simulink model "Solar_model2_AKhmad_Sameh"  (R2024b)
settings: Solver=FixedStepAuto  StartTime=0.0  StopTime=35000  FixedStep=1  RelTol=1e-3
settings Model: Creator=AKhmad  LastModifiedBy=AKhmad
settings OptimizationCC: ReuseModelBlockBuffer=off
settings RTWCC: GPUComputeCapability=3.5

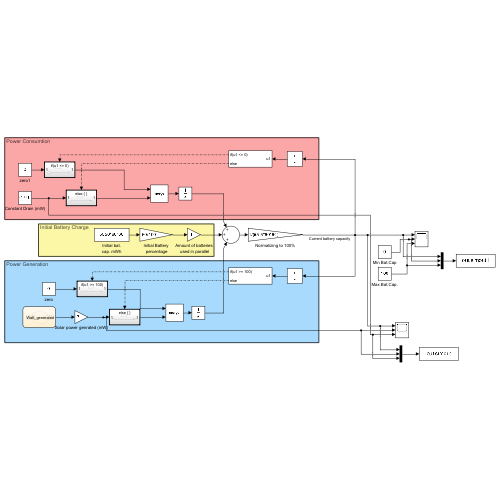
[thumbnail: Simulink's stored preview of the top-level diagram]
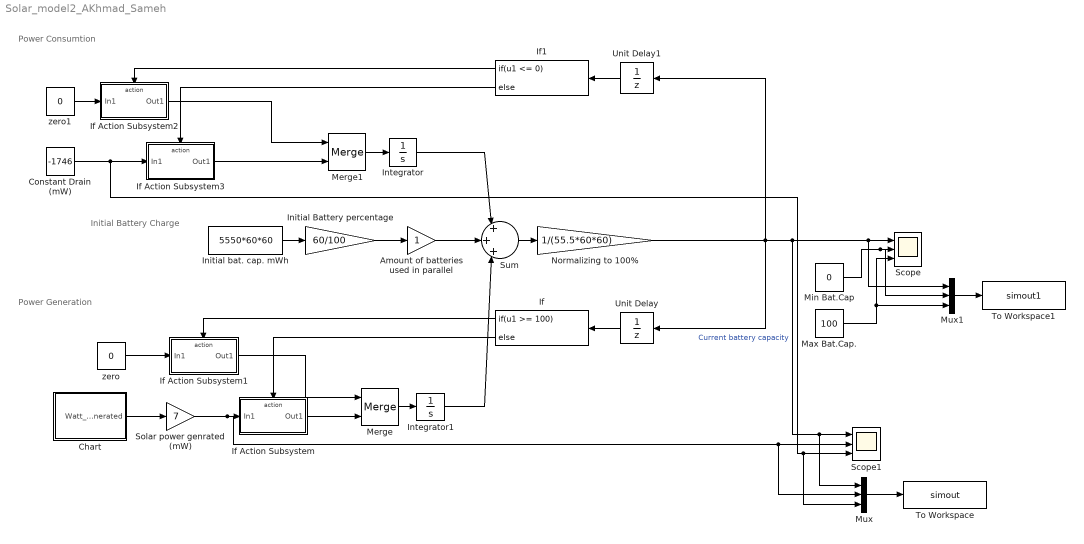
== system Solar_model2_AKhmad_Sameh ==
  note: Initial Battery Charge
  note: Power Generation
  note: Power Consumtion
  Amount of batteries used in parallel : Gain
  Chart : Stateflow chart  TreatAsAtomicUnit=on
  Constant Drain (mW) : Constant  Value=-1746
  If : If  IfExpression=u1 >= 100
  If Action Subsystem : Subsystem  TreatAsAtomicUnit=on
  If Action Subsystem1 : Subsystem  TreatAsAtomicUnit=on
  If Action Subsystem2 : Subsystem  TreatAsAtomicUnit=on
  If Action Subsystem3 : Subsystem  TreatAsAtomicUnit=on
  If1 : If  IfExpression=u1 <= 0
  Initial Battery percentage : Gain  Gain=60/100
  Initial bat. cap. mWh : Constant  Value=5550*60*60
  Integrator : Integrator
  Integrator1 : Integrator
  Max Bat.Cap. : Constant  Value=100
  Merge : Merge
  Merge1 : Merge
  Min Bat.Cap : Constant  Value=0
  Mux : Mux  Inputs=3
  Mux1 : Mux  Inputs=3
  Normalizing to 100% : Gain  Gain=1/(55.5*60*60)
  Scope : Scope  NumInputPorts=3
  Scope1 : Scope  NumInputPorts=3
  Solar power genrated (mW) : Gain  Gain=7
  Sum : Sum  Inputs=|+|+|+|  OutMin=0  OutMax=1
  To Workspace : ToWorkspace  VariableName=simout  SaveFormat=Timeseries  SampleTime=-1
  To Workspace1 : ToWorkspace  VariableName=simout1  SaveFormat=Timeseries  SampleTime=-1
  Unit Delay : UnitDelay  InitialCondition=100  SampleTime=-1  HasFrameUpgradeWarning=on
  Unit Delay1 : UnitDelay  InitialCondition=50  SampleTime=-1  HasFrameUpgradeWarning=on
  zero : Constant  Value=0
  zero1 : Constant  Value=0
  wires:
  Constant Drain (mW)/1 -> Mux/3, Scope1/3, If Action Subsystem3/1(In1)
  Integrator/1 -> Sum/1
  Chart/1(Watt_generated) -> Solar power genrated (mW)/1
  Sum/1 -> Normalizing to 100%/1
  Min Bat.Cap/1 -> Mux1/2, Scope/2
  Max Bat.Cap./1 -> Scope/3, Mux1/3
  Solar power genrated (mW)/1 -> Mux/2, Scope1/2, If Action Subsystem/1(In1)
  Initial bat. cap. mWh/1 -> Initial Battery percentage/1
  Amount of batteries used in parallel/1 -> Sum/2
  Normalizing to 100%/1 -> Mux/1, Scope1/1, Mux1/1, Scope/1, Unit Delay/1, Unit Delay1/1  "Current battery capacity"
  If/1 -> If Action Subsystem1/Action
  If Action Subsystem/1(Out1) -> Merge/2
  If/2 -> If Action Subsystem/Action
  If Action Subsystem1/1(Out1) -> Merge/1
  zero/1 -> If Action Subsystem1/1(In1)
  Merge/1 -> Integrator1/1
  Unit Delay/1 -> If/1
  Integrator1/1 -> Sum/3
  Unit Delay1/1 -> If1/1
  If Action Subsystem3/1(Out1) -> Merge1/2
  If1/1 -> If Action Subsystem2/Action
  If1/2 -> If Action Subsystem3/Action
  zero1/1 -> If Action Subsystem2/1(In1)
  Merge1/1 -> Integrator/1
  If Action Subsystem2/1(Out1) -> Merge1/1
  Initial Battery percentage/1 -> Amount of batteries used in parallel/1
  Mux/1 -> To Workspace/1
  Mux1/1 -> To Workspace1/1

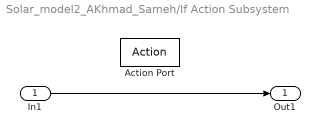
== system Solar_model2_AKhmad_Sameh/If Action Subsystem ==
  In1 : Inport
  Action Port : ActionPort  ActionPortLabel=else
  Out1 : Outport
  wires:
  In1/1 -> Out1/1

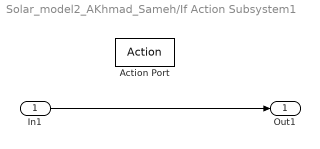
== system Solar_model2_AKhmad_Sameh/If Action Subsystem1 ==
  In1 : Inport
  Action Port : ActionPort  ActionPortLabel=if(u1 >= 100)
  Out1 : Outport
  wires:
  In1/1 -> Out1/1

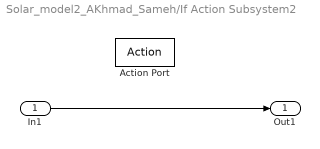
== system Solar_model2_AKhmad_Sameh/If Action Subsystem2 ==
  In1 : Inport
  Action Port : ActionPort  ActionPortLabel=if(u1 <= 0)
  Out1 : Outport
  wires:
  In1/1 -> Out1/1

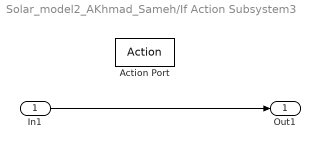
== system Solar_model2_AKhmad_Sameh/If Action Subsystem3 ==
  In1 : Inport
  Action Port : ActionPort  ActionPortLabel=else
  Out1 : Outport
  wires:
  In1/1 -> Out1/1

== stateflow chart Solar_model2_AKhmad_Sameh/Chart ==
  state in_the_sun
    entry:
    Watt_generated=5.4*60;
  state no_in_the_sun
    entry:
    Watt_generated=0;
  no_in_the_sun -> in_the_sun : after(2160,sec)
  (default) -> no_in_the_sun
  in_the_sun -> no_in_the_sun : after(3240,sec)
  data: Watt_generated output
